simulink model "mechanisation_quaternion"  (R2016b)
settings: Solver=ode15s  StartTime=0.0  StopTime=10.0  RelTol=10^-1  AbsTol=10^-1
undefined symbols (not defined in the file or in its folder): deg, rad, s
libraries: simulink x6, aerolibconvert2 x2, dspfdesign x1, dspsrcs4 x1, aerolib6dof2 x1
settings Model: Creator=liana  LastModifiedBy=liana
settings SolverCC: SolverJacobianMethodControl=SparsePerturbation  SolverResetMethod=Robust

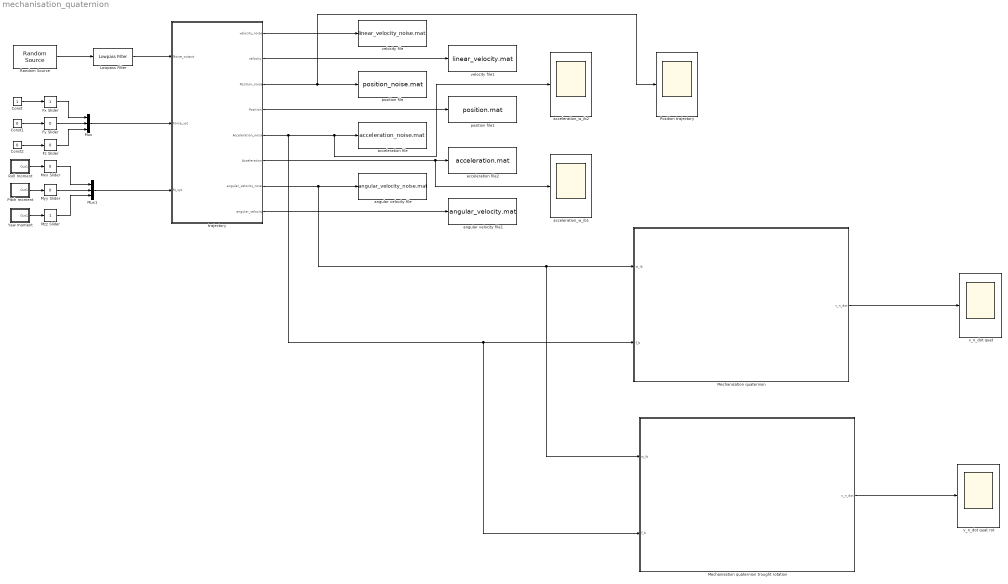
== system mechanisation_quaternion ==
  Const : Constant
  Const1 : Constant  Value=0
  Const2 : Constant  Value=0
  Fx Slider : simulink/Math Operations/Slider Gain  low=-1  gain=1  high=1
  Fy Slider : simulink/Math Operations/Slider Gain  low=-1  gain=0  high=1
  Fz Slider : simulink/Math Operations/Slider Gain  low=-1  gain=0  high=1
  Lowpass Filter : dspfdesign/Lowpass Filter  FilterType=FIR  DesignForMinimumOrder=on  FilterOrder=50  PassbandFrequency=8e3  StopbandFrequency=12e3  PassbandRipple=0.1  StopbandAttenuation=80  InheritSampleRate=off  SampleRate=44100  SimulateUsing=Interpreted execution  roundingMode=Floor  coeffsDataTypeStr=fixdt(1,16)
  Mechanisation quaternion : Subsystem
  Mechanisation quaternion trought rotation : Subsystem
  Mux : Mux  Inputs=3
  Mux1 : Mux  Inputs=3
  Mxx Slider : simulink/Math Operations/Slider Gain  low=0  gain=0  high=1
  Myy Slider : simulink/Math Operations/Slider Gain  low=0  gain=0  high=1
  Mzz Slider : simulink/Math Operations/Slider Gain  low=-1  gain=1  high=3
  Pitch moment : Subsystem  mask(timed input){t=[0 3 3 4 4 5 5  7.5 7.5 8.5 8.5 9.5 9.5 10], u=[0 0  1 1 -1 -1.005 0 0 -1 -1 1 1 0 0]*3.138/2}
      mask prompts: t "time values:"; u "input values"
      mask Display: plot(t,u)
  Position trajectory : Scope
  Random Source : dspsrcs4/Random Source  SrcType=Gaussian  NormMethod=Ziggurat  CltLength=12  MinVal=0  MaxVal=1  MeanVal=[0.05 0.05 0.05]'  VarVal=[5 5 5]'  RepMode=Not repeatable  rawSeed=1  IsInherit=off  SampMode=Discrete  SampTime=1  SampFrame=1  DataType=Double  OutComplex=Real  OutputFrames=off
  Roll moment : Subsystem  mask(timed input){t=[0 1 1 2 2  10], u=[1 1 -1 -.998  0 0]*3.144/2}
      mask prompts: t "time values:"; u "input values"
      mask Display: plot(t,u)
  Yaw moment : Subsystem  mask(timed input){t=[0 6 6 7 7 8 8 10], u=[0 0  -1 -1 1 1 0 0]*3.1/2}
      mask prompts: t "time values:"; u "input values"
      mask Display: plot(t,u)
  acceleration file : ToFile  Filename=acceleration_noise.mat  MatrixName=acc  SaveFormat=Timeseries
  acceleration file2 : ToFile  Filename=acceleration.mat  MatrixName=acc  SaveFormat=Timeseries
  acceleration_w_ib1 : Scope
  acceleration_w_ib2 : Scope
  angular velocity file : ToFile  Filename=angular_velocity_noise.mat  MatrixName=av  SaveFormat=Timeseries
  angular velocity file1 : ToFile  Filename=angular_velocity.mat  MatrixName=av  SaveFormat=Timeseries
  position file : ToFile  Filename=position_noise.mat  MatrixName=pos_noise  SaveFormat=Timeseries
  position file1 : ToFile  Filename=position.mat  MatrixName=pos  SaveFormat=Timeseries
  trajectory : Subsystem
  "v_n_dot quat " : Scope
  v_n_dot quat rot : Scope
  velocity file : ToFile  Filename=linear_velocity_noise.mat  MatrixName=lv  SaveFormat=Timeseries
  velocity file1 : ToFile  Filename=linear_velocity.mat  MatrixName=lv  SaveFormat=Timeseries
  wires:
  Mechanisation quaternion/1(v_n_dot) -> "v_n_dot quat "/1
  trajectory/5(Acceleration_noise) -> Mechanisation quaternion trought rotation/2(f_b), Mechanisation quaternion/2(f_b), acceleration_w_ib2/1, acceleration file/1
  Yaw moment/1(Out1) -> Mzz Slider/1
  Pitch moment/1(Out1) -> Myy Slider/1
  Roll moment/1(Out1) -> Mxx Slider/1
  Const2/1 -> Fz Slider/1
  Const1/1 -> Fy Slider/1
  Const/1 -> Fx Slider/1
  Mzz Slider/1 -> Mux1/3
  Myy Slider/1 -> Mux1/2
  Mxx Slider/1 -> Mux1/1
  Fy Slider/1 -> Mux/2
  Fz Slider/1 -> Mux/3
  Fx Slider/1 -> Mux/1
  Mux/1 -> trajectory/2(Force_xyz)
  Mux1/1 -> trajectory/3(M_xyz)
  trajectory/1(velocity_noise) -> velocity file/1
  trajectory/2(velocity) -> velocity file1/1
  trajectory/4(Position) -> position file1/1
  trajectory/6(Acceleration) -> acceleration_w_ib1/1, acceleration file2/1
  trajectory/8(angular_velocity) -> angular velocity file1/1
  trajectory/3(Position_noise) -> Position trajectory/1, position file/1
  trajectory/7(angular_velocity_noise) -> Mechanisation quaternion trought rotation/1(w_ib), Mechanisation quaternion/1(w_ib), angular velocity file/1
  Random Source/1 -> Lowpass Filter/1
  Lowpass Filter/1 -> trajectory/1(Noise_output)
  Mechanisation quaternion trought rotation/1(v_n_dot) -> v_n_dot quat rot/1

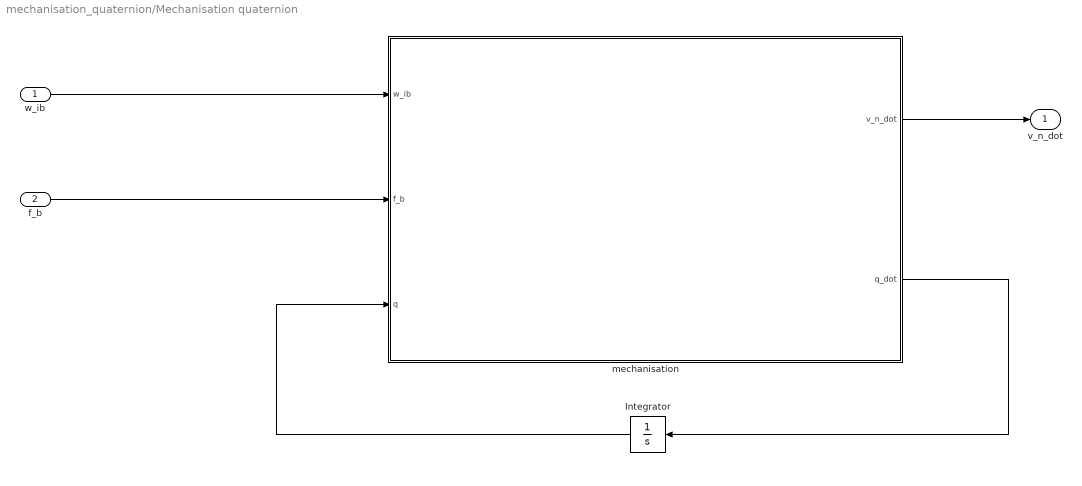
== system mechanisation_quaternion/Mechanisation quaternion ==
  w_ib : Inport
  f_b : Inport  Port=2
  Integrator : Integrator  InitialCondition=[1 0 0 0]  AbsoluteTolerance=10^-3
  mechanisation : MATLAB Function  TreatAsAtomicUnit=on
  v_n_dot : Outport
  wires:
  w_ib/1 -> mechanisation/1(w_ib)
  mechanisation/1(v_n_dot) -> v_n_dot/1
  mechanisation/2(q_dot) -> Integrator/1
  Integrator/1 -> mechanisation/3(q)
  f_b/1 -> mechanisation/2(f_b)

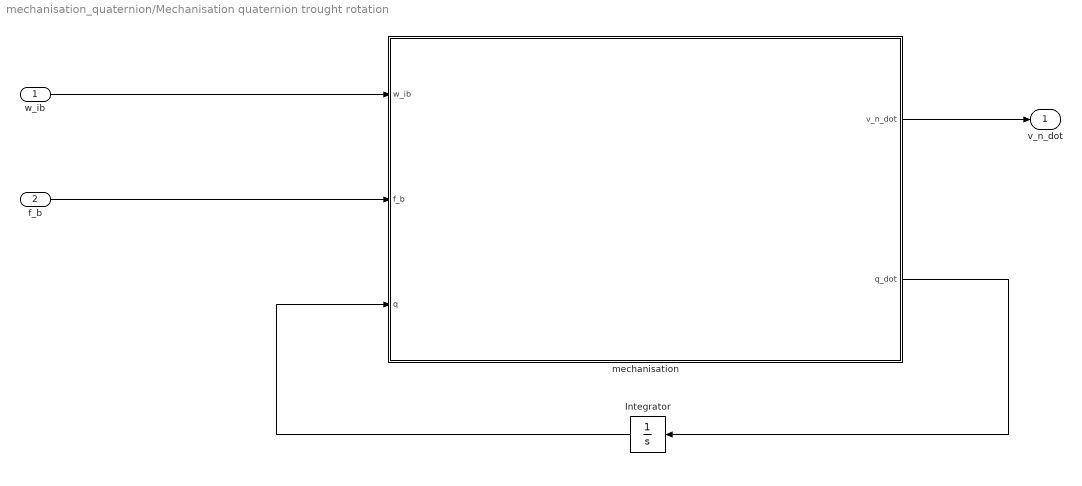
== system mechanisation_quaternion/Mechanisation quaternion trought rotation ==
  w_ib : Inport
  f_b : Inport  Port=2
  Integrator : Integrator  InitialCondition=[1 0 0 0]  AbsoluteTolerance=10^-3
  mechanisation : MATLAB Function  TreatAsAtomicUnit=on
  v_n_dot : Outport
  wires:
  w_ib/1 -> mechanisation/1(w_ib)
  mechanisation/1(v_n_dot) -> v_n_dot/1
  mechanisation/2(q_dot) -> Integrator/1
  Integrator/1 -> mechanisation/3(q)
  f_b/1 -> mechanisation/2(f_b)

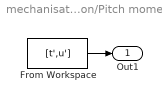
== system mechanisation_quaternion/Pitch moment ==
  From Workspace : FromWorkspace  VariableName=[t',u']  SampleTime=0
  Out1 : Outport
  wires:
  From Workspace/1 -> Out1/1

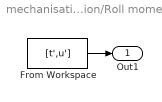
== system mechanisation_quaternion/Roll moment ==
  From Workspace : FromWorkspace  VariableName=[t',u']  SampleTime=0
  Out1 : Outport
  wires:
  From Workspace/1 -> Out1/1

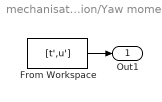
== system mechanisation_quaternion/Yaw moment ==
  From Workspace : FromWorkspace  VariableName=[t',u']  SampleTime=0
  Out1 : Outport
  wires:
  From Workspace/1 -> Out1/1

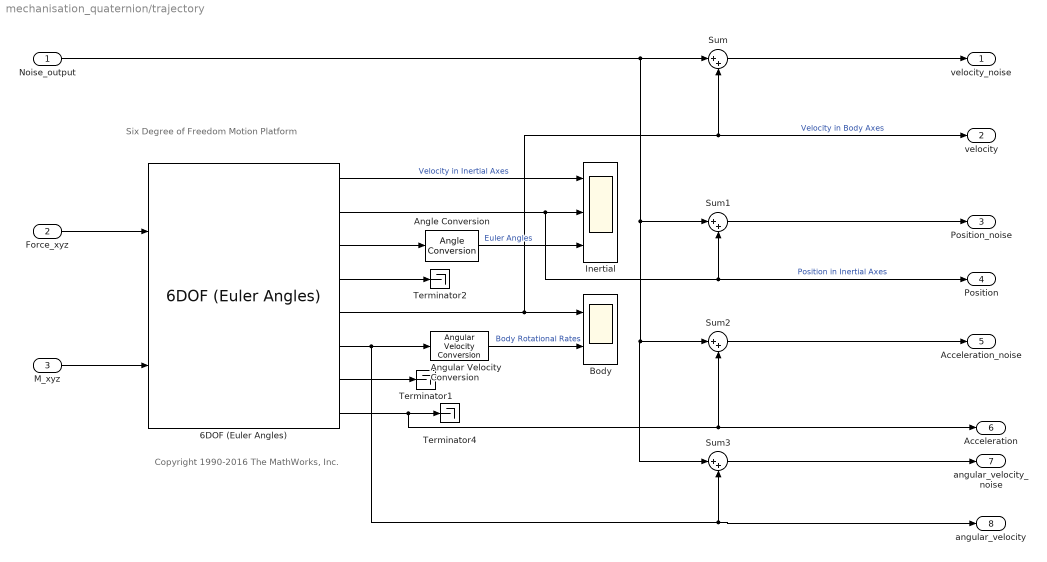
== system mechanisation_quaternion/trajectory ==
  note: Six Degree of Freedom Motion Platform
  note: Copyright 1990-2016 The MathWorks, Inc.
  Noise_output : Inport
  Force_xyz : Inport  Port=2
  M_xyz : Inport  Port=3
  6DOF (Euler Angles) : aerolib6dof2/6DOF (Euler Angles)  units=Metric (MKS)  mtype=Fixed  rep=Euler Angles  xme_0=[0 0 0]  Vm_0=[0 0 0]  eul_0=[0 0 0]  pm_0=[0 0 0]  mass_0=1.0  mass_e=0.5  mass_f=2.0  inertia=eye(3)  inertia_e=eye(3)  inertia_f=2*eye(3)  k_quat=1.0  vre_flag=on
  Angle Conversion : aerolibconvert2/Angle Conversion  IU=rad  OU=deg
  Angular Velocity Conversion : aerolibconvert2/Angular Velocity Conversion  IU=rad/s  OU=deg/s
  Body : Scope  NumInputPorts=2
  Inertial : Scope  NumInputPorts=3
  Sum{,1..3} (4 alike) : Sum  Inputs=|++
  Terminator1 : Terminator
  Terminator2 : Terminator
  Terminator4 : Terminator
  velocity_noise : Outport
  velocity : Outport  Port=2
  Position_noise : Outport  Port=3
  Position : Outport  Port=4
  Acceleration_noise : Outport  Port=5
  Acceleration : Outport  Port=6
  angular_velocity_noise : Outport  Port=7
  angular_velocity : Outport  Port=8
  wires:
  6DOF (Euler Angles)/8 -> Sum2/2, Acceleration/1, Terminator4/1
  Sum/1 -> velocity_noise/1
  Noise_output/1 -> Sum3/1, Sum2/1, Sum1/1, Sum/1
  6DOF (Euler Angles)/3 -> Angle Conversion/1
  6DOF (Euler Angles)/5 -> Sum/2, velocity/1, Body/1  "Velocity in Body Axes"
  Sum3/1 -> angular_velocity_noise/1
  Force_xyz/1 -> 6DOF (Euler Angles)/1
  Sum1/1 -> Position_noise/1
  6DOF (Euler Angles)/6 -> angular_velocity/1, Sum3/2, Angular Velocity Conversion/1
  Angular Velocity Conversion/1 -> Body/2  "Body Rotational Rates"
  6DOF (Euler Angles)/7 -> Terminator1/1
  6DOF (Euler Angles)/2 -> Position/1, Sum1/2, Inertial/2  "Position in Inertial Axes"
  6DOF (Euler Angles)/4 -> Terminator2/1
  Sum2/1 -> Acceleration_noise/1
  Angle Conversion/1 -> Inertial/3  "Euler Angles"
  6DOF (Euler Angles)/1 -> Inertial/1  "Velocity in Inertial Axes"
  M_xyz/1 -> 6DOF (Euler Angles)/2

== matlab function mechanisation_quaternion/Mechanisation quaternion trought rotation/mechanisation ==
  data: w_ib input; f_b input; v_n_dot output; q_dot output; q input
function [v_n_dot, q_dot] = mechanisation(w_ib, f_b, q)

% q = [w x y z]
q=q'; %from col to row vector

g_n = [0 0 9.81]';


Skew = skew(w_ib);

R_nb = quat2rotm(q);

v_n_dot = R_nb * f_b + g_n;
R_nb_dot = Skew * R_nb;

q_dot = rotm2quat(R_nb_dot);

== matlab function mechanisation_quaternion/Mechanisation quaternion/mechanisation ==
  data: w_ib input; f_b input; v_n_dot output; q_dot output; q input
function [v_n_dot, q_dot] = mechanisation(w_ib, f_b, q)

% q = [w x y z]
q=q'; %from col to row vector

g_n = [0 0 9.81]';

%old implementation

% Skew = skew(w_ib);
% 
% R_nb = quat2rotm(q);
% 
% v_n_dot = R_nb * f_b + g_n;
% R_nb_dot = Skew * R_nb;


R_nb = quat2rotm(q);
v_n_dot = R_nb * f_b + g_n;

E = [ -q(2)  q(1) -q(4)  q(3);
      -q(3)  q(4)  q(1) -q(2);
      -q(4)  q(3) -q(2)  q(1)];

q_dot = (1/2)*E'*w_ib;
